simulink model "lab3task2"  (R2021a)
settings: Solver=VariableStepAuto  StartTime=0.0  StopTime=10.0  RelTol=1e-3
libraries: simulink x2, dsparch4 x1, commsynccomp2 x1
settings Model: Creator=youssefashraf  LastModifiedBy=youssefashraf

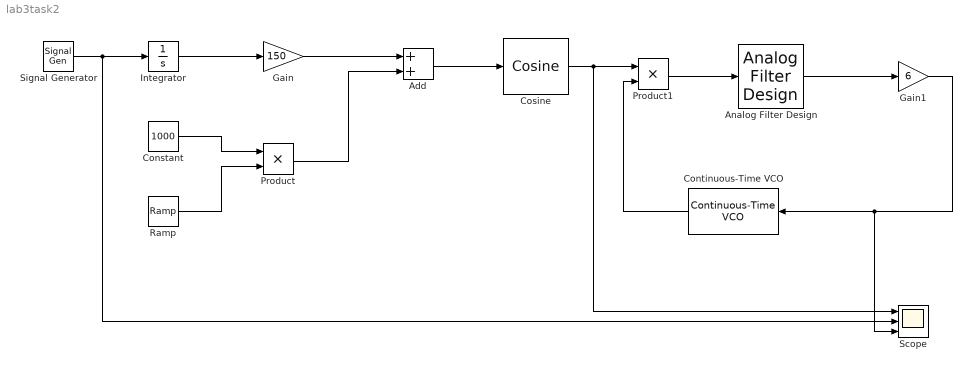
== system lab3task2 ==
  Add : Sum
  Analog Filter Design : dsparch4/Analog Filter Design  method=Butterworth  filttype=Lowpass  N=8  Wlo=630  Whi=80  Rp=2  Rs=40
  Constant : Constant  Value=1000
  Continuous-Time VCO : commsynccomp2/Continuous-Time VCO  Ac=1  Fc=1000  Kc=1  Ph=0
      settings: SourceProductBaseCode=CM
  Cosine : simulink/Lookup Tables/Cosine  Formula=cos(2*pi*u)  NumDataPoints=(2^5)+1  OutputWordLength=16  InternalRulePriority=Speed
      settings: SourceProductBaseCode=SL
  Gain : Gain  Gain=150
  Gain1 : Gain  Gain=6
  Integrator : Integrator
  Product : Product
  Product1 : Product
  Ramp : simulink/Sources/Ramp  slope=1  start=0  InitialOutput=0
  Scope : Scope  NumInputPorts=3
  Signal Generator : SignalGenerator  Amplitude=2  Frequency=100
  wires:
  Signal Generator/1 -> Scope/2, Integrator/1
  Integrator/1 -> Gain/1
  Constant/1 -> Product/1
  Ramp/1 -> Product/2
  Gain/1 -> Add/1
  Product/1 -> Add/2
  Add/1 -> Cosine/1
  Cosine/1 -> Scope/1, Product1/1
  Product1/1 -> Analog Filter Design/1
  Analog Filter Design/1 -> Gain1/1
  Continuous-Time VCO/1 -> Product1/2
  Gain1/1 -> Continuous-Time VCO/1, Scope/3
